simulink model "ModifiedBatteryModel1"  (R2019a)
settings: Solver=VariableStepAuto  StartTime=0.0  StopTime=10.0  RelTol=1e-3
libraries: fl_lib x5, nesl_utility x5
settings Model: Creator=nikos  LastModifiedBy=nikos

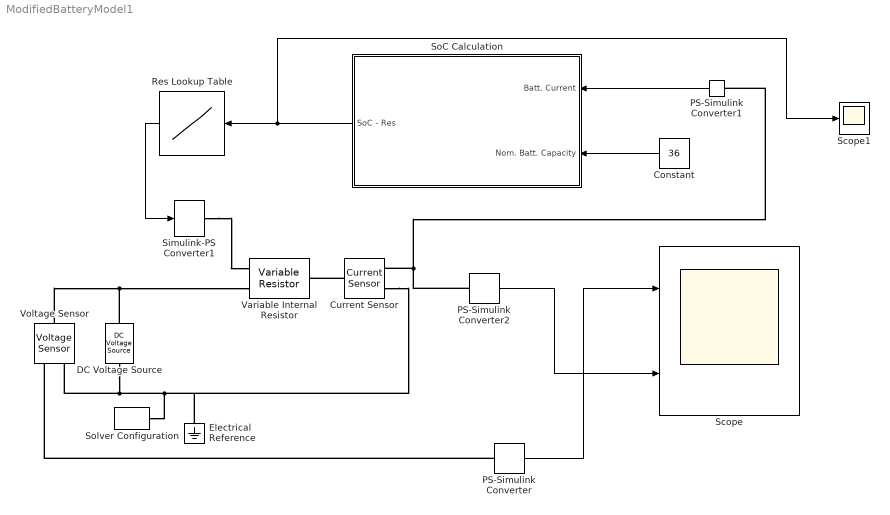
== system ModifiedBatteryModel1 ==
  Constant : Constant  Value=36
  Current Sensor : fl_lib/Electrical/Electrical Sensors/Current Sensor
  DC Voltage Source : fl_lib/Electrical/Electrical Sources/DC Voltage Source  v0=72 V
  Electrical Reference : fl_lib/Electrical/Electrical Elements/Electrical Reference
  PS-Simulink Converter : nesl_utility/PS-Simulink Converter  PhysicalDomain=network_engine_domain  SubClassName=ps_output  LeftPortType=input  RightPortType=output  PseudoPeriodic=off  Frequencies=[]  Unit=1  AffineConversion=off
  PS-Simulink Converter1 : nesl_utility/PS-Simulink Converter  PhysicalDomain=network_engine_domain  SubClassName=ps_output  LeftPortType=input  RightPortType=output  PseudoPeriodic=off  Frequencies=[]  Unit=1  AffineConversion=off
  PS-Simulink Converter2 : nesl_utility/PS-Simulink Converter  PhysicalDomain=network_engine_domain  SubClassName=ps_output  LeftPortType=input  RightPortType=output  PseudoPeriodic=off  Frequencies=[]  Unit=1  AffineConversion=off
  Res Lookup Table : Lookup_n-D  NumberOfTableDimensions=1  BreakpointsForDimension1=[0, 10, 20, 30, 40, 50, 60, 70, 80, 90, 100]  Table=[0.011448, 0.011038, 0.011281, 0.011236, 0.010959, 0.010714, 0.010698, 0.010712, 0.010917, 0.011304, 0.011603]  InternalRulePriority=Speed  RndMeth=Simplest  InputSameDT=on
  Scope : Scope  NumInputPorts=2
  Scope1 : Scope
  Simulink-PS Converter1 : nesl_utility/Simulink-PS Converter  PhysicalDomain=network_engine_domain  SubClassName=ps_input  LeftPortType=input  RightPortType=output  PseudoPeriodic=off  Frequencies=[]  NoiseDistribution=none  NoiseParameters=[]  Unit=1  AffineConversion=off  FilteringAndDerivatives=zero  SimscapeFilterOrder=1  InputFilterTimeConstant=0.001  UdotUserProvided=1
  SoC Calculation : Subsystem
  Solver Configuration : nesl_utility/Solver Configuration  PhysicalDomain=network_engine_domain  SubClassName=solver  LeftPortType=input  RightPortType=generic  Tones=[]  Harmonics=[]  SimulateNoise=off  Profile=off  UseLocalSampling=off  EnableSwitchedLinearOptims=on  FrequencyDomain=off  UseCCode=off  RelTol=0.001  AbsTol=1e-06  MinStep=1e-09  ToWorkspace=off  RevertToSquareIcSolve=off  NumHomotopyIterations=100  PhasorMode=off  PhasorModeNumHarmonics=1  DoDC=off  ResidualTolerance=1e-09  UseLocalSolver=off  LocalSolverChoice=NE_BACKWARD_EULER_ADVANCER  LocalSolverSampleTime=0.001  DoFixedCost=off  MaxNonlinIter=3  MaxModeIter=2  LinearAlgebra=Sparse  EquationFormulation=NE_TIME_EF  DelaysMemoryBudget=1024  AutomaticFiltering=on  FilteringTimeConstant=0.001  PartitionStorageMethod=AS_NEEDED  PartitionMemoryBudget=1024  PartitionMethod=FAST
  Variable Internal Resistor : fl_lib/Electrical/Electrical Elements/Variable Resistor  Rmin=1 Ohm  i_specify=off  i_priority=High  i=0 A  i_nominal_specify=off  i_nominal_unit=A  i_nominal_value=1  v_specify=off  v_priority=High  v=0 V  v_nominal_specify=off  v_nominal_unit=V  v_nominal_value=1
  Voltage Sensor : fl_lib/Electrical/Electrical Sensors/Voltage Sensor
  wires:
  PS-Simulink Converter1/1 -> SoC Calculation/1("Batt. Current ")
  Constant/1 -> SoC Calculation/2("Nom. Batt. Capacity ")
  SoC Calculation/1(SoC - Res) -> Scope1/1, Res Lookup Table/1
  Res Lookup Table/1 -> Simulink-PS Converter1/1
  PS-Simulink Converter2/1 -> Scope/2
  PS-Simulink Converter/1 -> Scope/1
  connections:
  Voltage Sensor/LConn1 -- DC Voltage Source/LConn1 -- Variable Internal Resistor/LConn2
  DC Voltage Source/RConn1 -- Solver Configuration/RConn1 -- Electrical Reference/LConn1 -- Current Sensor/RConn2 -- Voltage Sensor/RConn2
  PS-Simulink Converter2/LConn1 -- PS-Simulink Converter1/LConn1 -- Current Sensor/RConn1
  Simulink-PS Converter1/RConn1 -- Variable Internal Resistor/LConn1
  PS-Simulink Converter/LConn1 -- Voltage Sensor/RConn1
  Current Sensor/LConn1 -- Variable Internal Resistor/RConn1

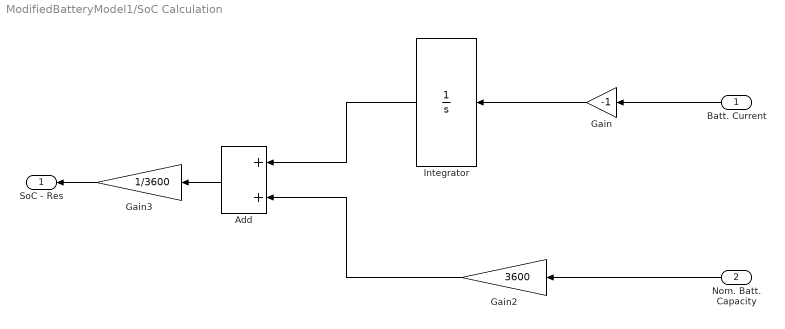
== system ModifiedBatteryModel1/SoC Calculation ==
  "Batt. Current " : Inport
  "Nom. Batt. Capacity " : Inport  Port=2  OutMin=0  OutMax=100
  Add : Sum
  Gain : Gain  Gain=-1
  Gain2 : Gain  Gain=3600
  Gain3 : Gain  Gain=1/3600
  Integrator : Integrator
  SoC - Res : Outport
  wires:
  Gain3/1 -> SoC - Res/1
  Integrator/1 -> Add/1
  Add/1 -> Gain3/1
  Gain2/1 -> Add/2
  "Nom. Batt. Capacity "/1 -> Gain2/1
  Gain/1 -> Integrator/1
  "Batt. Current "/1 -> Gain/1
